simulink model "apll"  (R2019b)
settings: Solver=VariableStepAuto  StartTime=0.0  StopTime=10  RelTol=1e-6  AbsTol=1e-6
values from neighbouring files (symbols this model uses):
  G_0 = db2mag(94)    [apll_attr.m]    (also in apll_const.m = db2mag(90.8); main.m = db2mag(g); test.m = db2mag(87.3))
  omega_0 = 0    [apll_attr.m]    (also in apll_const.m; main.m = 700; test.m)
  tau_p1 = 1.65*1e-3    (= 0.00165)    [apll_attr.m]    (also in apll_attr_nondim_1.m; apll_attr_nondim_2.m; apll_attr_nondim_3.m; apll_const.m)
  tau_p2 = 1.65*1e-3    (= 0.00165)    [apll_attr.m]    (also in apll_attr_nondim_1.m; apll_attr_nondim_2.m; apll_attr_nondim_3.m; apll_const.m)
  tau_z1 = 165*1e-6    (= 0.000165)    [apll_attr.m]    (also in apll_attr_nondim_1.m; apll_attr_nondim_2.m; apll_attr_nondim_3.m; apll_const.m)
  tau_z2 = 165*1e-6    (= 0.000165)    [apll_attr.m]    (also in apll_attr_nondim_1.m; apll_attr_nondim_2.m; apll_attr_nondim_3.m; apll_const.m)
libraries: simulink x1
settings Model: Creator=Elena  LastModifiedBy=Elena

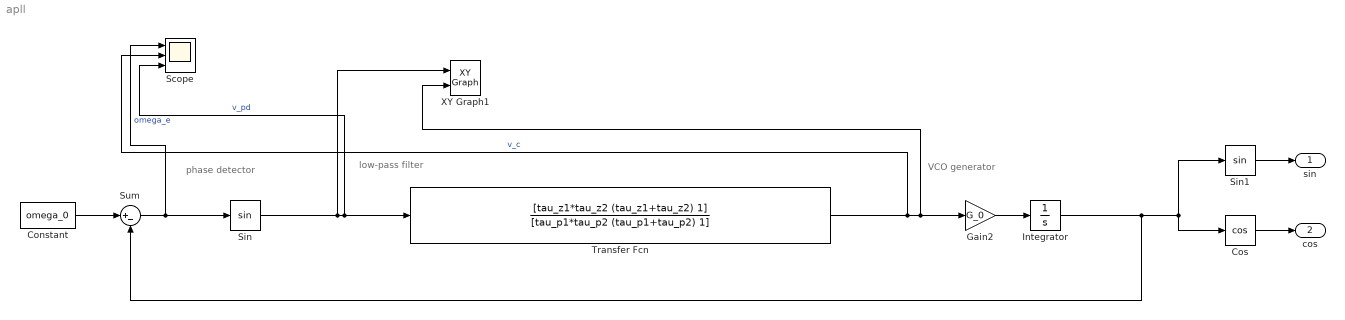
== system apll ==
  note: VCO generator
  note: phase detector
  note: low-pass filter
  Constant : Constant  Value=omega_0
  Cos : Trigonometry  Operator=cos
  Gain2 : Gain  Gain=G_0
  Integrator : Integrator  InitialCondition=pi/6
  Scope : Scope  NumInputPorts=3
  Sin : Trigonometry
  Sin1 : Trigonometry
  Sum : Sum  Inputs=|+-
  Transfer Fcn : TransferFcn  Numerator=[tau_z1*tau_z2 (tau_z1+tau_z2) 1]  Denominator=[tau_p1*tau_p2 (tau_p1+tau_p2) 1]
  XY Graph1 : simulink/Sinks/XY Graph  xmin=-1  xmax=1  ymin=-1  ymax=1  st=-1
  sin : Outport
  cos : Outport  Port=2
  wires:
  Sum/1 -> Scope/1, Sin/1  "omega_e"
  Cos/1 -> cos/1
  Transfer Fcn/1 -> Scope/2, XY Graph1/2, Gain2/1  "v_c"
  Sin1/1 -> sin/1
  Sin/1 -> XY Graph1/1, Scope/3, Transfer Fcn/1  "v_pd"
  Gain2/1 -> Integrator/1
  Integrator/1 -> Sin1/1, Cos/1, Sum/2
  Constant/1 -> Sum/1
